simulink model "Task5"  (R2024a)
settings: Solver=VariableStepAuto  StartTime=0.0  StopTime=100.0  RelTol=1e-3
settings Model: Creator=artemzmailov  LastModifiedBy=artemzmailov

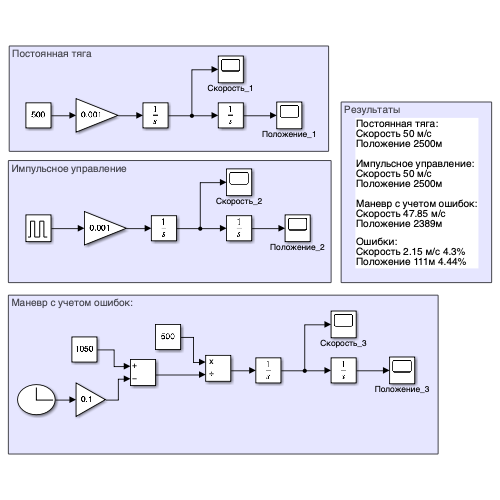
[thumbnail: Simulink's stored preview of the top-level diagram]
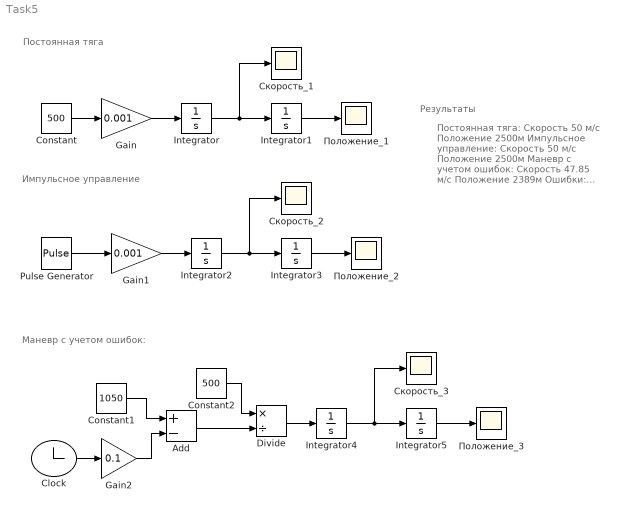
== system Task5 ==
  note: Результаты
  note: Постоянная тяга:
      | Скорость 50 м/c
      | Положение 2500м
      |
      | Импульсное управление:
      | Скорость 50 м/c
      | Положение 2500м
      |
      | Маневр с учетом ошибок:
      | Скорость 47.85 м/c
      | Положение 2389м
      |
      | Ошибки:
      | Скорость 2.15 м/c 4.3%
      | Положение 111м 4.44%
  note: Маневр с учетом ошибок:
  note: Импульсное управление
  note: Постоянная тяга
  Add : Sum  Inputs=+-
  Clock : Clock
  Constant : Constant  Value=500
  Constant1 : Constant  Value=1050
  Constant2 : Constant  Value=500
  Divide : Product  Inputs=*/
  Gain : Gain  Gain=0.001
  Gain1 : Gain  Gain=0.001
  Gain2 : Gain  Gain=0.1
  Integrator{,1..5} (6 alike) : Integrator
  Pulse Generator : DiscretePulseGenerator  PulseType=Time based  Amplitude=500  Period=200  PulseWidth=50
  Положение_1 : Scope
  Положение_2 : Scope
  Положение_3 : Scope
  Скорость_1 : Scope
  Скорость_2 : Scope
  Скорость_3 : Scope
  wires:
  Constant/1 -> Gain/1
  Gain/1 -> Integrator/1
  Integrator/1 -> Integrator1/1, Скорость_1/1
  Integrator1/1 -> Положение_1/1
  Pulse Generator/1 -> Gain1/1
  Integrator3/1 -> Положение_2/1
  Gain1/1 -> Integrator2/1
  Integrator2/1 -> Integrator3/1, Скорость_2/1
  Clock/1 -> Gain2/1
  Constant1/1 -> Add/1
  Gain2/1 -> Add/2
  Add/1 -> Divide/2
  Constant2/1 -> Divide/1
  Integrator5/1 -> Положение_3/1
  Integrator4/1 -> Integrator5/1, Скорость_3/1
  Divide/1 -> Integrator4/1
